simulink model "power_3phsignalseq"  (Simulink 6.0)
settings: Solver=ode23tb  SolverMode=SingleTasking  StartTime=0.0  StopTime=0.2  MaxStep=5e-5  RelTol=1e-3  AbsTol=1e-2
libraries: powerlib x6, powerlib_extras x2
settings Model: Creator=sybille  LastModifiedBy=batserve  ExtModeTrigMode=oneshot  ExtModeArmWhenConnect=off  ExtModeAutoUpdateStatusClock=off  ProdHWDeviceType=Specified
settings DataIOCC: Decimation=10  LimitDataPoints=off  SaveFinalState=on  SaveOutput=off  SignalLoggingName=sigsOut
settings OptimizationCC: BlockReduction=off  BooleanDataType=off
settings DebuggingCC: CheckExecutionContextPreStartOutputMsg=on  CheckExecutionContextRuntimeOutputMsg=on  SolverPrmCheckMsg=none  UnconnectedInputMsg=none  UnconnectedOutputMsg=none
settings HardwareCC: ProdBitPerShort=32  ProdBitPerInt=16  ProdHWDeviceType=Specified  TargetUnknown=on
settings RTWCC: TemplateMakefile=grt_vc.tmf

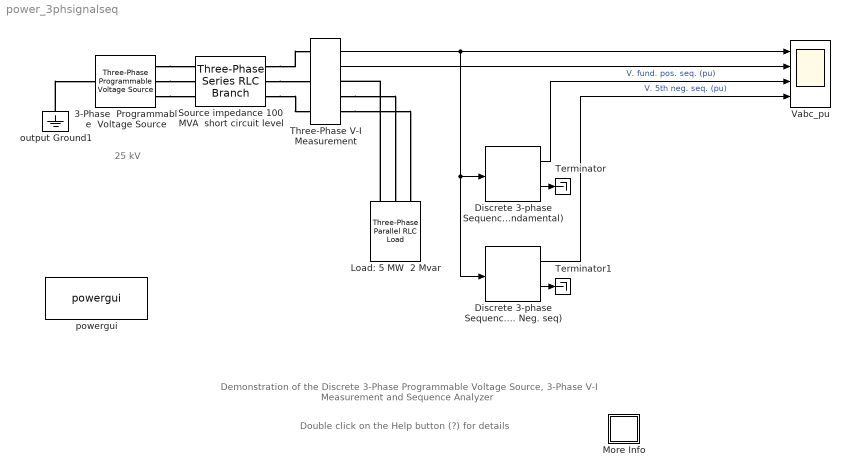
== system power_3phsignalseq ==
  note: Demonstration of the Discrete 3-Phase Programmable Voltage Source,
      |  3-Phase V-I Measurement and Sequence Analyzer
  note: Double click on the Help button (?) for details
  note: 25 kV
  3-Phase  Programmable  Voltage Source : powerlib/Electrical Sources/Three-Phase Programmable Voltage Source  PositiveSequence="[25e3 0  60]"  VariationEntity=Amplitude  VariationType=Step  VariationStep=0.5  VariationRate=10  VariationMagnitude=0.3  VariationFrequency=2  VariationTiming=[0.05 1]  VariationPhaseA=off  Amplitudes=[1 0.8 1.2 1.0]  TimeValues=[0 0.1 0.15 0.2]  HarmonicGeneration=on  HarmonicA=[5 0.08 -45 2]  HarmonicB=[2 0 0 2]  Timing="[0.1  1]"
  Discrete 3-phase Sequence Analyzer (5th harm. Neg. seq) : powerlib_extras/Discrete Measurements/Discrete 3-phase Sequence Analyzer  Freq=60  n=5  seq=Negative  Par_Init=[0 0]  Ts=50e-6
  Discrete 3-phase Sequence Analyzer (Fundamental) : powerlib_extras/Discrete Measurements/Discrete 3-phase Sequence Analyzer  Freq=60  n=1  seq=Positive  Par_Init=[0 0]  Ts=50e-6
  Load: 5 MW  2 Mvar : powerlib/Elements/Three-Phase Parallel RLC Load  Orientation=down  PhysicalDomain=powersysdomain  SubClassName=unknown  LeftPortType=p1  RightPortType=p1  LConnTagsString=A|B|C  Configuration=Y (grounded)  NominalVoltage=25e3  NominalFrequency=60  ActivePower=5e6  InductivePower=0  CapacitivePower=2e6  Measurements=None
  More Info : Subsystem
      mask Display: disp('?')
  Source impedance 100 MVA  short circuit level : powerlib/Elements/Three-Phase Series RLC Branch  PhysicalDomain=powersysdomain  SubClassName=unknown  LeftPortType=p1  RightPortType=p1  LConnTagsString=A|B|C  RConnTagsString=A|B|C  Resistance=25^2/100/10  Inductance=25^2/100/377  Capacitance=inf  Measurements=None
  Terminator : Terminator
  Terminator1 : Terminator
  Three-Phase V-I Measurement : powerlib/Measurements/Three-Phase V-I Measurement  VoltageMeasurement=phase-to-ground  SetLabelV=off  LabelV=V1  Vpu=on  Vbase=25e3  CurrentMeasurement=yes  SetLabelI=off  LabelI=I1  Ipu=on  Pbase=10e6  OutputType=Magnitude  PhasorSimulation=off  PSBequivalent=0
  Vabc_pu : Scope  NumInputPorts=4
      settings: TimeRange=0.2  YMin=-2~-2~0~0  YMax=2~1~2~0.2  DataFormat=Array  SampleInput=on
  output Ground1 : powerlib/Elements/Ground  Orientation=down  PhysicalDomain=powersysdomain  SubClassName=unknown  LeftPortType=p1  RightPortType=p1  LConnTagsString=a
  powergui : powerlib/powergui  Priority=2  Frange=[0:2:500]  Ylog=off  Xlog=off  save=off  variable=ZData  ZoomFFT=on  StartTime=0.0  cycles=1  DisplayStyle=off  fundamental=60  FreqAxis=off  MaxFrequency=1000  frequencyindice=1  frequencyindicesteady=1  RmsSteady=1  display=off  Ts=50e-6  methode=off  frequency=60  echomessages=off
  wires:
  Discrete 3-phase Sequence Analyzer (Fundamental)/1 -> Vabc_pu/3  "V. fund. pos. seq. (pu)"
  Discrete 3-phase Sequence Analyzer (5th harm. Neg. seq)/1 -> Vabc_pu/4  "V. 5th neg. seq. (pu)"
  Discrete 3-phase Sequence Analyzer (Fundamental)/2 -> Terminator/1
  Discrete 3-phase Sequence Analyzer (5th harm. Neg. seq)/2 -> Terminator1/1
  Three-Phase V-I Measurement/2 -> Vabc_pu/2
  Three-Phase V-I Measurement/1 -> Vabc_pu/1, Discrete 3-phase Sequence Analyzer (Fundamental)/1, Discrete 3-phase Sequence Analyzer (5th harm. Neg. seq)/1
  connections:
  Source impedance 100 MVA  short circuit level/RConn1 -- Three-Phase V-I Measurement/LConn1
  Source impedance 100 MVA  short circuit level/RConn2 -- Three-Phase V-I Measurement/LConn2
  Source impedance 100 MVA  short circuit level/RConn3 -- Three-Phase V-I Measurement/LConn3
  3-Phase  Programmable  Voltage Source/RConn1 -- Source impedance 100 MVA  short circuit level/LConn1
  3-Phase  Programmable  Voltage Source/RConn2 -- Source impedance 100 MVA  short circuit level/LConn2
  3-Phase  Programmable  Voltage Source/RConn3 -- Source impedance 100 MVA  short circuit level/LConn3
  output Ground1/LConn1 -- 3-Phase  Programmable  Voltage Source/LConn1
  Load: 5 MW  2 Mvar/LConn1 -- Three-Phase V-I Measurement/RConn1
  Three-Phase V-I Measurement/RConn2 -- Load: 5 MW  2 Mvar/LConn2
  Three-Phase V-I Measurement/RConn3 -- Load: 5 MW  2 Mvar/LConn3

== system power_3phsignalseq/More Info ==
  note: Circuit Description
  note: This demonstration ilustrates use of the 3-Phase Programmable Voltage Source,
      | 3-Phase V-I Measurement, and Sequence Analyzer blocks
  note: A  25kV, 100 MVA short-circuit level,  equivalent network feeds a 5MW, 2 Mvar capacitive load.
      |
      | The internal voltage of the source is controlled by the Discrete 3-phase Programmable Voltage Source block.
      |
      | Open the source dialog box and look at the parameters controlling the voltage. A positive-sequence of
      | 1.0 pu, 0 degrees is specified. At t = 0.05 s a step of 0.5 pu is applied on positive-sequence voltage magnitude,
      | then, at t = 0.1 s, 0.08 pu of 5th harmonic in negative sequence is added on the 1.5 pu voltage.
      |
      | In order to start simulation in steady state, the three voltage sources are initialized  with a
      | positive-sequence voltage of 25 kV, 0 degree, 60 Hz.
      |
      | The Three-Phase V-I Measurement block allows to monitor the three load voltages and currents.
      | Open its dialog box and see how this block allows to output the voltages and currents in pu.
      |
      | Two Discrete 3-phase Sequence Analyzer blocks are used to monitor the positive-sequeence of the three fundamental voltages Va, Vb, Vc
      | and the negative-sequence component of the 5th harmonic.
      |
      | The whole system, (power network, programmable source, and sequence analyzers) is discretized at a 50 us sample time.
  note: Demonstration
  note: Choose  Simulation/Start and observe the  voltage and current waveforms.
      |
      | The simulation starts in steady state with 1 pu voltage.
      | At t = 0.05 sec, the internal voltage is increased to 1.5 pu. At t = 0.10 sec. 0.08 pu of 5th harmonic internal voltage is added.
      |
      | Observe the fundamental component (pos. seq.) and the 5th harmonic component  (neg. seq.) measured by the two sequence analyzers.
      | The 0.08 pu 5th harmonic internal voltage is amplified at 0.14 pu at the load terminals.
      | As the sequence analyzers use Fourier analysis, their response time is one cycle.
  note: G. Sybille (Hydro-Quebec)
